simulink model "CalculateOptimalFlux"  (R2025b)
settings: Solver=FixedStepDiscrete  StartTime=0.0  StopTime=10.0  RelTol=1e-3
model workspace (MAT data in the model file):
  Gain_I_flux = Simulink.Parameter
  Gain_I_flux.Value = 0.25
  Gain_I_flux.Complexity = 'real'
  Gain_I_flux.Dimensions = [1 1]
  Gain_I_flux.DataType = 'auto'
  Gain_P_flux = Simulink.Parameter
  Gain_P_flux.Value = 0.5
  Gain_P_flux.Complexity = 'real'
  Gain_P_flux.Dimensions = [1 1]
  Gain_P_flux.DataType = 'auto'
undefined symbols (not defined in the file): DiscIntNeverNeededParam
settings Model: DataDictionary=TractionEmotorSoftwareArchInterfaceData.sldd  Creator=dakaihu  LastModifiedBy=dakaihu
settings OptimizationCC: DefaultParameterBehavior=Inlined  GainParamInheritBuiltInType=on  UseFloatMulNetSlope=on  InlineInvariantSignals=on  PassReuseOutputArgsAs=Individual arguments  ZeroExternalMemoryAtStartup=off  ZeroInternalMemoryAtStartup=off  NoFixptDivByZeroProtection=on  EfficientFloat2IntCast=on  LifeSpan=1  OptimizeBlockOrder=speed  DifferentSizesBufferReuse=on  EfficientTunableParamExpr=on
settings DebuggingCC: ParameterTunabilityLossMsg=error
settings HardwareCC: ProdBitPerChar=16.0  ProdBitPerInt=16.0  ProdBitPerPointer=32.0  ProdBitPerSizeT=32.0  ProdBitPerPtrDiffT=32.0  ProdLargestAtomicInteger=Integer  ProdLargestAtomicFloat=None  ProdWordSize=16.0  ProdLongLongMode=on  ProdHWDeviceType=Texas Instruments->C2000
settings SFSimCC: MATLABDynamicMemAlloc=off
settings RTWCC: SystemTargetFile=ert.tlc  TemplateMakefile=ert_default_tmf  Description=Embedded Coder
settings CodeAppCC: ForceParamTrailComments=on  IgnoreCustomStorageClasses=off  MaxIdLength=60.0  OperatorAnnotations=on  SimulinkDataObjDesc=on  SFDataObjDesc=on  CustomSymbolStrGlobalVar=rt$N$M  CustomSymbolStrType=$N$M  CustomSymbolStrFcn=$N$M$F  CustomSymbolStrMacro=$N$M  InsertBlockDesc=on
settings ERTTargetCC: ERTCustomFileTemplate=example_file_process.tlc  ERTFilePackagingFormat=CompactWithDataFile  TargetLangStandard=C99 (ISO)  GenerateSampleERTMain=on  IncludeMdlTerminateFcn=off  CombineSignalStateStructs=on  SuppressErrorStatus=on  SupportAbsoluteTime=off  SupportComplex=off

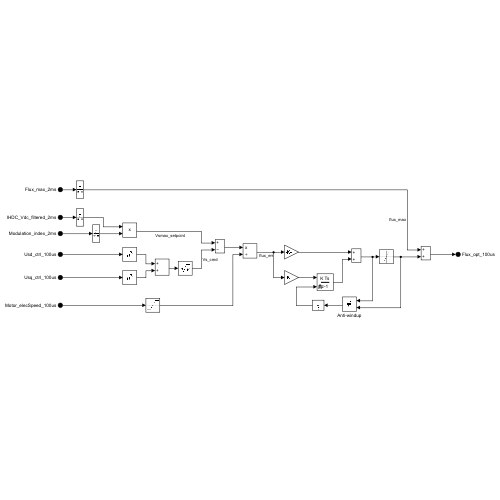
[thumbnail: Simulink's stored preview of the top-level diagram]
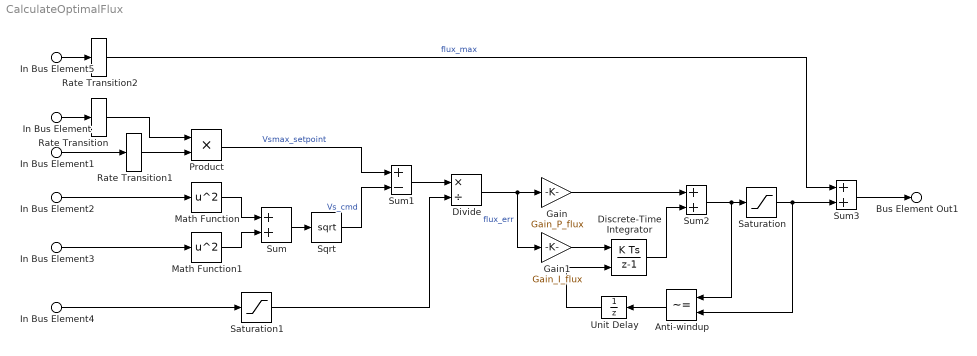
== system CalculateOptimalFlux ==
  In Bus Element : Inport  PortName=IHDC_Vdc_filtered_2ms
  In Bus Element1 : Inport  Port=2  PortName=Modulation_index_2ms
  In Bus Element2 : Inport  Port=3  PortName=Usd_ctrl_100us
  In Bus Element3 : Inport  Port=4  PortName=Usq_ctrl_100us
  In Bus Element4 : Inport  Port=5  PortName=Motor_elecSpeed_100us
  In Bus Element5 : Inport  Port=6  PortName=Flux_max_2ms
  Anti-windup : RelationalOperator  Operator=~=  OutDataTypeStr=boolean  RndMeth=Simplest  InputSameDT=off
  Discrete-Time Integrator : DiscreteIntegrator  ExternalReset=level  SampleTime=-1  ICPrevOutput=DiscIntNeverNeededParam  ICPrevScaledInput=DiscIntNeverNeededParam
  Divide : Product  Inputs=*/
  Gain : Gain  Gain=Gain_P_flux
  Gain1 : Gain  Gain=Gain_I_flux
  Math Function : Math  Operator=square
  Math Function1 : Math  Operator=square
  Product : Product
  Rate Transition : RateTransition  Deterministic=off
  Rate Transition1 : RateTransition  Deterministic=off
  Rate Transition2 : RateTransition  Deterministic=off
  Saturation : Saturate  UpperLimit=0.005  LowerLimit=-0.005
  Saturation1 : Saturate  UpperLimit=inf  LowerLimit=0.1
  Sqrt : Sqrt
  Sum : Sum
  Sum1 : Sum  Inputs=+-
  Sum2 : Sum
  Sum3 : Sum
  Unit Delay : UnitDelay  SampleTime=-1  HasFrameUpgradeWarning=on
  Bus Element Out1 : Outport  PortName=Flux_opt_100us
  wires:
  In Bus Element2/1 -> Math Function/1
  In Bus Element3/1 -> Math Function1/1
  Sum/1 -> Sqrt/1
  Math Function/1 -> Sum/1
  Math Function1/1 -> Sum/2
  In Bus Element1/1 -> Rate Transition1/1
  Product/1 -> Sum1/1  "Vsmax_setpoint"
  Sqrt/1 -> Sum1/2  "Vs_cmd"
  Sum1/1 -> Divide/1
  Divide/1 -> Gain1/1, Gain/1  "flux_err"
  Gain1/1 -> Discrete-Time Integrator/1
  Gain/1 -> Sum2/1
  Discrete-Time Integrator/1 -> Sum2/2
  Sum2/1 -> Anti-windup/1, Saturation/1
  Anti-windup/1 -> Unit Delay/1
  Unit Delay/1 -> Discrete-Time Integrator/2
  Saturation/1 -> Sum3/2, Anti-windup/2
  In Bus Element5/1 -> Rate Transition2/1
  Sum3/1 -> Bus Element Out1/1
  In Bus Element/1 -> Rate Transition/1
  Rate Transition/1 -> Product/1
  Rate Transition1/1 -> Product/2
  Rate Transition2/1 -> Sum3/1  "flux_max"
  In Bus Element4/1 -> Saturation1/1
  Saturation1/1 -> Divide/2
